simulink model "tGeminiTaskPlannerHarness"  (R2026a)
settings: Solver=FixedStepDiscrete  StopTime=0.1  FixedStep=0.1
PreLoadFcn:
  | addpath(fileparts(fileparts(which(bdroot)))); robotSimParams;
undefined symbols (not defined in the file or in its folder): GeminiERPlan, tGTP_depth, tGTP_image
settings Model: Creator=smaddina  LastModifiedBy=smaddina

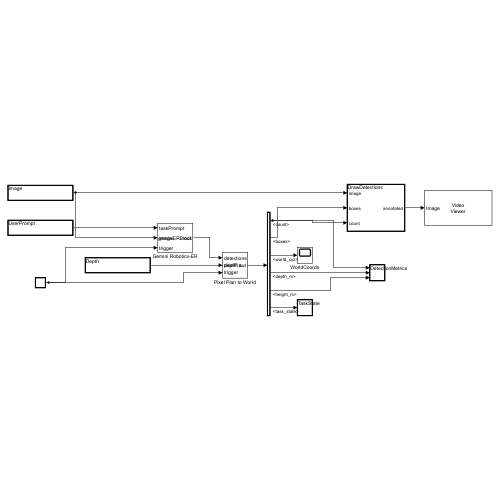
[thumbnail: Simulink's stored preview of the top-level diagram]
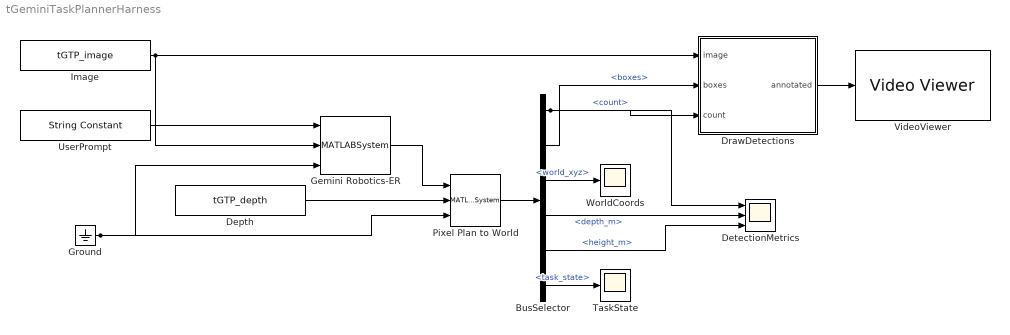
== system tGeminiTaskPlannerHarness ==
  BusSelector : BusSelector  OutputSignals=count,boxes,world_xyz,depth_m,height_m,task_state
  Depth : Constant  Value=tGTP_depth  VectorParams1D=off  SampleTime=0.1
  DetectionMetrics : Scope  NumInputPorts=3
  DrawDetections : MATLAB Function  TreatAsAtomicUnit=on
  Gemini Robotics-ER : MATLABSystem  System=geminiERBlock  UseEnvApiKey=on  Mode=GeminiERPlan('MaxDetections', 8, 'ApplyMask', false)  ScenarioPrompt=|  ThinkingBudget=0
      | You are guiding a robot arm that performs intelligent bin picking.
      | 
      | Scene layout (overhead camera looking straight down):
      | - A rectangular bin in the centre of the image holds unsorted white plastic pipe fittings.
      | - A flat work table to the LEFT of the bin is a placement target.
      | - A flat work table to the RIGHT of the bin is a placement target.
      | - A robot arm (may appear at the image edges) performs the pick-and-place.
      | 
      | The objects in the bin are white plastic pipe fittings of four types:
      | - Cross fitting  (X-shape): four-way connector, four symmetric arms in a plus pattern.
      | - Tee fitting    (T-shape): three-way connector, one straight channel with one perpendicular branch.
      | - Elbow fitting  (L-shape): two-way connector bent 90 degrees.
      | - Straight fitting (I-shape): cylindrical straight-through connector, no bends.
      mask Type: geminiERBlock
  Ground : Ground
  Image : Constant  Value=tGTP_image  VectorParams1D=off  OutDataTypeStr=uint8  SampleTime=0.1
  Pixel Plan to World : MATLABSystem  System=pixelPlanToWorldBlock  FocalLength=750  PrincipalPoint=[640 360]  CameraLoc=[0.5 0 1.5]  CameraRot=pi/2*ones([1 3])  MaxBinDistance=0.95  DropHeightOffset=0.1  RobotOffsetZ=0.625001  MaxDetections=8
      mask Type: pixelPlanToWorldBlock
  TaskState : Scope
  UserPrompt : StringConstant  String="\"\""
  VideoViewer : VideoViewer  FigPos=[1 1030 1920 933]
  WorldCoords : Scope
  wires:
  Image/1 -> DrawDetections/1(image), Gemini Robotics-ER/2
  BusSelector/1 -> DrawDetections/3(count), DetectionMetrics/1  "<count>"
  BusSelector/4 -> DetectionMetrics/2  "<depth_m>"
  BusSelector/5 -> DetectionMetrics/3  "<height_m>"
  BusSelector/3 -> WorldCoords/1  "<world_xyz>"
  BusSelector/6 -> TaskState/1  "<task_state>"
  BusSelector/2 -> DrawDetections/2(boxes)  "<boxes>"
  DrawDetections/1(annotated) -> VideoViewer/1
  UserPrompt/1 -> Gemini Robotics-ER/1
  Gemini Robotics-ER/1 -> Pixel Plan to World/1
  Ground/1 -> Pixel Plan to World/3, Gemini Robotics-ER/3
  Depth/1 -> Pixel Plan to World/2
  Pixel Plan to World/1 -> BusSelector/1

== matlab function tGeminiTaskPlannerHarness/DrawDetections ==
  data: image input; annotated output; boxes input; count input
function annotated = DrawDetections(image, boxes, count)
%#codegen
coder.extrinsic('insertShape');
annotated = image;
n = floor(min(double(count), 8));
if n > 0
    rects = zeros(n, 4);
    for i = 1:n
        b = boxes(i,:);  %% [y_min x_min y_max x_max]
        rects(i,:) = [b(2), b(1), b(4)-b(2), b(3)-b(1)];
    end
    annotated = insertShape(image, 'Rectangle', rects, 'Color', 'green', 'LineWidth', 3);
end
